simulink model "Controller"  (R2018b)
settings: configuration reference "control_config" (kept outside this file)
values from neighbouring files (symbols this model uses):
  CONTROL_EXPORT = Simulink.Parameter(CONTROL_EXPORT_VALUE)    [controller_model_init.m]
  CONTROL_PARAM = Simulink.Parameter(CONTROL_PARAM_VALUE)    [controller_model_init.m]
undefined symbols (not defined in the file or in its folder): actuator_cmd, CONTROL_CONST, CONTROL_PARAM_VALUE, ControlMode, DiscIntNeverNeededParam, phi_cmd, theta_cmd, timestamp, w_cmd
libraries: simulink x38, FMT_Model_Lib x20
(part 2 of 3)

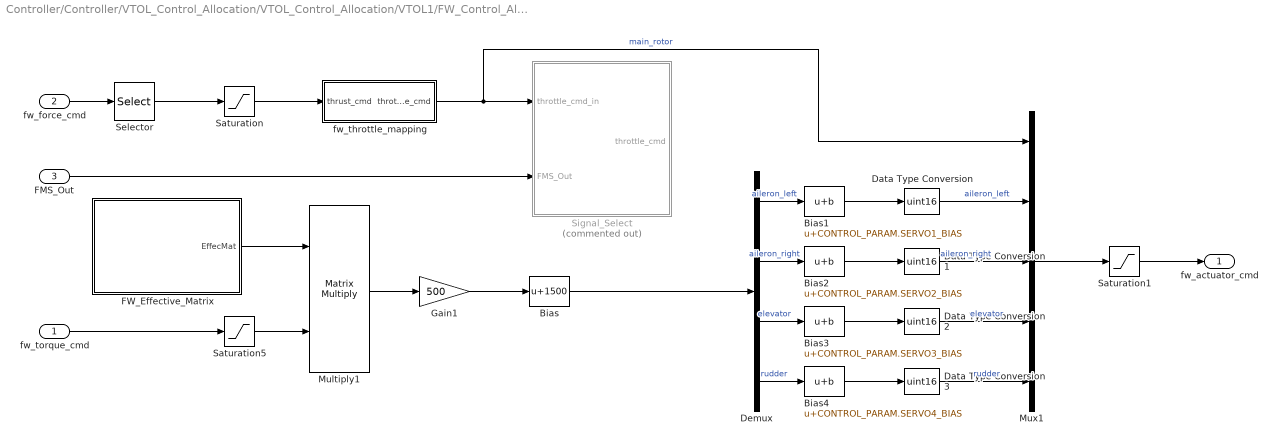
== system Controller/Controller/VTOL_Control_Allocation/VTOL_Control_Allocation/VTOL1/FW_Control_Allocation ==
  fw_torque_cmd : Inport
  fw_force_cmd : Inport  Port=2
  FMS_Out : Inport  Port=3
  Bias : Bias  Bias=1500
  Bias1 : Bias  Bias=CONTROL_PARAM.SERVO1_BIAS
  Bias2 : Bias  Bias=CONTROL_PARAM.SERVO2_BIAS
  Bias3 : Bias  Bias=CONTROL_PARAM.SERVO3_BIAS
  Bias4 : Bias  Bias=CONTROL_PARAM.SERVO4_BIAS
  Data Type Conversion{,1..3} (4 alike) : DataTypeConversion  OutDataTypeStr=uint16
  Demux : Demux
  FW_Effective_Matrix : Subsystem
  Gain1 : Gain  Gain=500  OutDataTypeStr=Inherit: Same as input  ParamDataTypeStr=Inherit: Same as input
  Multiply1 : Product  Multiplication=Matrix(*)  OutDataTypeStr=Inherit: Same as first input
  Mux1 : Mux  Inputs=5
  Saturation : Saturate  UpperLimit=1  LowerLimit=0
  Saturation1 : Saturate  UpperLimit=up_limit  LowerLimit=lo_limit  OutDataTypeStr=uint16
  Saturation5 : Saturate  UpperLimit=1  LowerLimit=-1
  Selector : Selector  InputPortWidth=3  IndexOptions=Index vector (dialog)  Indices=1  OutputSizes=1
  Signal_Select : Subsystem  Commented=on
  fw_throttle_mapping : Subsystem
  fw_actuator_cmd : Outport
  wires:
  Data Type Conversion/1 -> Mux1/2  "aileron_left"
  Gain1/1 -> Bias/1
  Saturation5/1 -> Multiply1/2
  Saturation/1 -> fw_throttle_mapping/1(thrust_cmd)
  Selector/1 -> Saturation/1
  Data Type Conversion1/1 -> Mux1/3  "aileron_right"
  Data Type Conversion3/1 -> Mux1/5  "rudder"
  FW_Effective_Matrix/1(EffecMat) -> Multiply1/1
  fw_force_cmd/1 -> Selector/1
  Data Type Conversion2/1 -> Mux1/4  "elevator"
  Mux1/1 -> Saturation1/1
  Multiply1/1 -> Gain1/1
  fw_torque_cmd/1 -> Saturation5/1
  fw_throttle_mapping/1(throttle_cmd) -> Mux1/1, Signal_Select/1(throttle_cmd_in)  "main_rotor"
  FMS_Out/1 -> Signal_Select/2(FMS_Out)
  Bias/1 -> Demux/1
  Saturation1/1 -> fw_actuator_cmd/1
  Bias2/1 -> Data Type Conversion1/1
  Bias1/1 -> Data Type Conversion/1
  Bias3/1 -> Data Type Conversion2/1
  Bias4/1 -> Data Type Conversion3/1
  Demux/1 -> Bias1/1  "aileron_left"
  Demux/2 -> Bias2/1  "aileron_right"
  Demux/3 -> Bias3/1  "elevator"
  Demux/4 -> Bias4/1  "rudder"

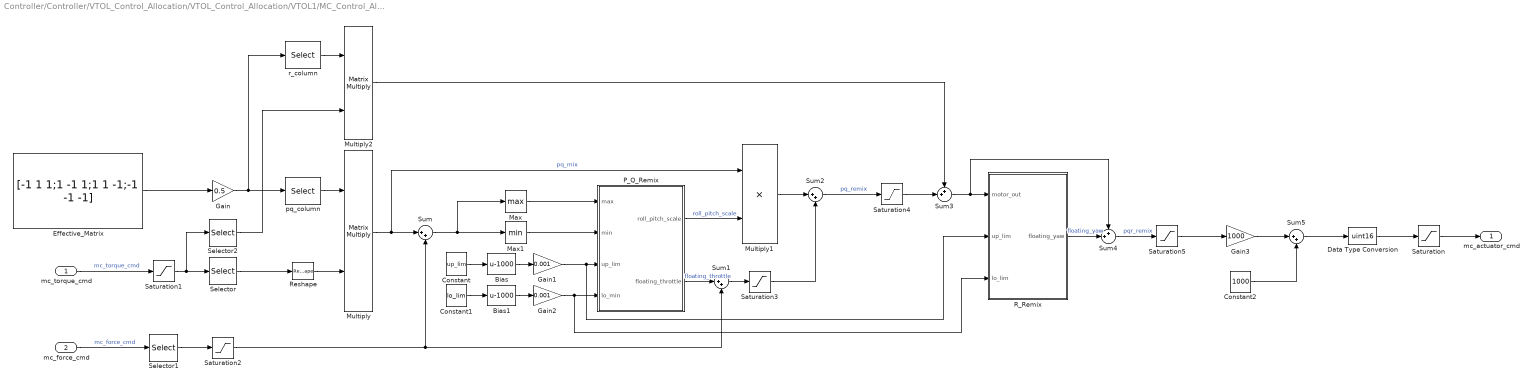
== system Controller/Controller/VTOL_Control_Allocation/VTOL_Control_Allocation/VTOL1/MC_Control_Allocation ==
  mc_torque_cmd : Inport
  mc_force_cmd : Inport  Port=2
  Bias : Bias  Bias=-1000
  Bias1 : Bias  Bias=-1000
  Constant : Constant  Value=up_lim  OutDataTypeStr=single
  Constant1 : Constant  Value=lo_lim  OutDataTypeStr=single
  Constant2 : Constant  Value=1000  OutDataTypeStr=uint32
  Data Type Conversion : DataTypeConversion  OutDataTypeStr=uint16
  Effective_Matrix : Constant  Value=[-1 1 1;1 -1 1;1 1 -1;-1 -1 -1]  OutDataTypeStr=single
  Gain : Gain  Gain=0.5
  Gain1 : Gain  Gain=0.001
  Gain2 : Gain  Gain=0.001
  Gain3 : Gain  Gain=1000  OutDataTypeStr=uint32
  Max : MinMax  Function=max
  Max1 : MinMax
  Multiply : Product  Multiplication=Matrix(*)  OutDataTypeStr=single
  Multiply1 : Product  OutDataTypeStr=single
  Multiply2 : Product  Multiplication=Matrix(*)  OutDataTypeStr=single
  P_Q_Remix : Subsystem
  R_Remix : MATLAB Function  TreatAsAtomicUnit=on
  Reshape : Reshape  OutputDimensionality=Column vector (2-D)
  Saturation : Saturate  UpperLimit=up_lim  LowerLimit=lo_lim
  Saturation1 : Saturate  UpperLimit=1  LowerLimit=-1
  Saturation{2..5} (4 alike) : Saturate  UpperLimit=1  LowerLimit=0
  Selector : Selector  InputPortWidth=3  IndexOptions=Index vector (dialog)  Indices=[1 2]  OutputSizes=1
  Selector1 : Selector  InputPortWidth=3  IndexOptions=Index vector (dialog)  Indices=3  OutputSizes=1
  Selector2 : Selector  InputPortWidth=3  IndexOptions=Index vector (dialog)  Indices=3  OutputSizes=1
  Sum{,1..2,5} (4 alike) : Sum  Inputs=|++
  Sum3 : Sum  Inputs=++|
  Sum4 : Sum  Inputs=++|
  pq_column : Selector  NumberOfDimensions=2  InputPortWidth=3  IndexOptions=Index vector (dialog),Index vector (dialog)  Indices=[1:4],[1 2]  OutputSizes=1,1
  r_column : Selector  NumberOfDimensions=2  InputPortWidth=3  IndexOptions=Index vector (dialog),Index vector (dialog)  Indices=[1:4],3  OutputSizes=1,1
  mc_actuator_cmd : Outport
  wires:
  Multiply/1 -> Multiply1/1, Sum/1  "pq_mix"
  Effective_Matrix/1 -> Gain/1
  mc_force_cmd/1 -> Selector1/1  "mc_force_cmd"
  Sum/1 -> Max/1, Max1/1
  Saturation/1 -> mc_actuator_cmd/1
  Reshape/1 -> Multiply/2
  Selector/1 -> Reshape/1
  Saturation1/1 -> Selector2/1, Selector/1
  Selector1/1 -> Saturation2/1
  pq_column/1 -> Multiply/1
  Max/1 -> P_Q_Remix/1(max)
  Max1/1 -> P_Q_Remix/2(min)
  Gain/1 -> r_column/1, pq_column/1
  P_Q_Remix/2(floating_throttle) -> Sum1/1  "floating_throttle"
  Sum1/1 -> Saturation3/1
  P_Q_Remix/1(roll_pitch_scale) -> Multiply1/2  "roll_pitch_scale"
  Multiply1/1 -> Sum2/1
  Saturation3/1 -> Sum2/2
  Sum2/1 -> Saturation4/1  "pq_remix"
  r_column/1 -> Multiply2/1
  Selector2/1 -> Multiply2/2
  Multiply2/1 -> Sum3/1
  Saturation4/1 -> Sum3/2
  Sum3/1 -> Sum4/1, R_Remix/1(motor_out)
  Constant/1 -> Bias/1
  Constant1/1 -> Bias1/1
  R_Remix/1(floating_yaw) -> Sum4/2  "floating_yaw"
  Sum4/1 -> Saturation5/1  "pqr_remix"
  Data Type Conversion/1 -> Saturation/1
  Bias/1 -> Gain1/1
  Gain1/1 -> P_Q_Remix/3(up_lim), R_Remix/2(up_lim)
  Bias1/1 -> Gain2/1
  Gain2/1 -> P_Q_Remix/4(lo_min), R_Remix/3(lo_lim)
  mc_torque_cmd/1 -> Saturation1/1  "mc_torque_cmd"
  Sum5/1 -> Data Type Conversion/1
  Saturation5/1 -> Gain3/1
  Gain3/1 -> Sum5/1
  Constant2/1 -> Sum5/2
  Saturation2/1 -> Sum1/2, Sum/2

== system Controller/Controller/VTOL_Control_Allocation/VTOL_Control_Allocation/VTOL1/MC_Control_Allocation1 ==
  mc_torque_cmd : Inport
  mc_force_cmd : Inport  Port=2
  Add : Sum  OutDataTypeStr=uint16
  Effective_Matrix : Constant  Value=[-sqrt(2) sqrt(2) 1;sqrt(2) -sqrt(2) 1;sqrt(2) sqrt(2) -1;-sqrt(2) -sqrt(2) -1]  OutDataTypeStr=single
  Gain : Gain  Gain=1000  OutDataTypeStr=Inherit: Same as input
  Multiply : Product  Multiplication=Matrix(*)  OutDataTypeStr=Inherit: Same as first input
  Saturation : Saturate  UpperLimit=1900  LowerLimit=1100
  Saturation1 : Saturate  UpperLimit=1  LowerLimit=-1
  Saturation2 : Saturate  UpperLimit=1  LowerLimit=0
  Selector1 : Selector  InputPortWidth=3  IndexOptions=Index vector (dialog)  Indices=3  OutputSizes=1
  throttle_mapping : Subsystem
  mc_actuator_cmd : Outport
  wires:
  throttle_mapping/1(throttle_cmd) -> Add/2
  Saturation2/1 -> throttle_mapping/1(thrust_cmd)
  Multiply/1 -> Gain/1  "tt2"
  mc_torque_cmd/1 -> Saturation1/1
  Saturation1/1 -> Multiply/2
  Selector1/1 -> Saturation2/1
  Gain/1 -> Add/1
  Effective_Matrix/1 -> Multiply/1
  mc_force_cmd/1 -> Selector1/1
  Add/1 -> Saturation/1
  Saturation/1 -> mc_actuator_cmd/1

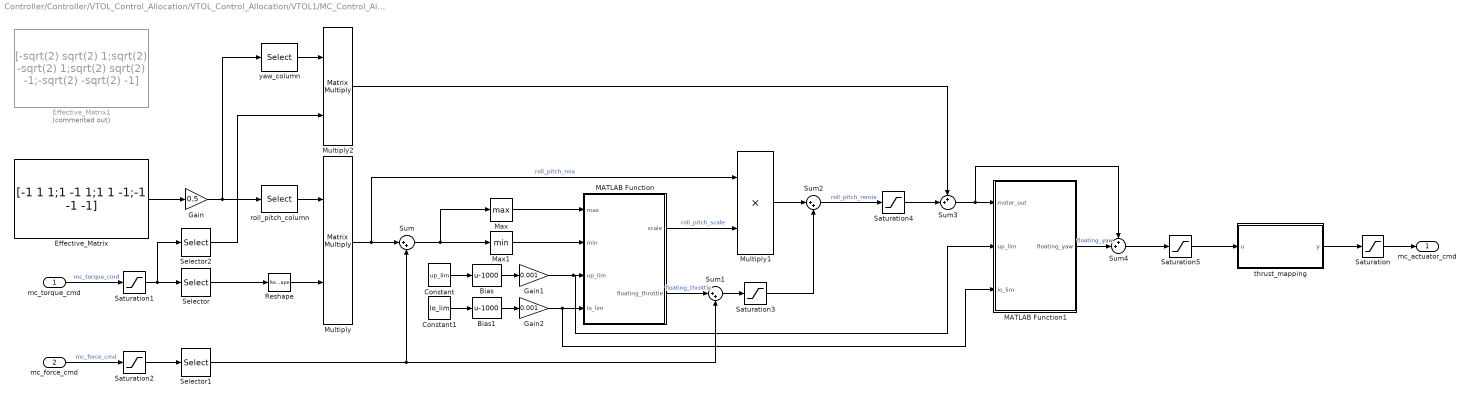
== system Controller/Controller/VTOL_Control_Allocation/VTOL_Control_Allocation/VTOL1/MC_Control_Allocation2 ==
  mc_torque_cmd : Inport
  mc_force_cmd : Inport  Port=2
  Bias : Bias  Bias=-1000
  Bias1 : Bias  Bias=-1000
  Constant : Constant  Value=up_lim  OutDataTypeStr=single
  Constant1 : Constant  Value=lo_lim  OutDataTypeStr=single
  Effective_Matrix : Constant  Value=[-1 1 1;1 -1 1;1 1 -1;-1 -1 -1]  OutDataTypeStr=single
  Effective_Matrix1 : Constant  Commented=on  Value=[-sqrt(2) sqrt(2) 1;sqrt(2) -sqrt(2) 1;sqrt(2) sqrt(2) -1;-sqrt(2) -sqrt(2) -1]  OutDataTypeStr=single
  Gain : Gain  Gain=0.5
  Gain1 : Gain  Gain=0.001
  Gain2 : Gain  Gain=0.001
  MATLAB Function : MATLAB Function  TreatAsAtomicUnit=on
  MATLAB Function1 : MATLAB Function  TreatAsAtomicUnit=on
  Max : MinMax  Function=max
  Max1 : MinMax
  Multiply : Product  Multiplication=Matrix(*)  OutDataTypeStr=Inherit: Same as first input
  Multiply1 : Product
  Multiply2 : Product  Multiplication=Matrix(*)  OutDataTypeStr=Inherit: Same as first input
  Reshape : Reshape  OutputDimensionality=Column vector (2-D)
  Saturation : Saturate  UpperLimit=up_lim  LowerLimit=lo_lim
  Saturation1 : Saturate  UpperLimit=1  LowerLimit=-1
  Saturation{2..5} (4 alike) : Saturate  UpperLimit=1  LowerLimit=0
  Selector : Selector  InputPortWidth=3  IndexOptions=Index vector (dialog)  Indices=[1 2]  OutputSizes=1
  Selector1 : Selector  InputPortWidth=3  IndexOptions=Index vector (dialog)  Indices=3  OutputSizes=1
  Selector2 : Selector  InputPortWidth=3  IndexOptions=Index vector (dialog)  Indices=3  OutputSizes=1
  Sum : Sum  Inputs=|++
  Sum1 : Sum  Inputs=|++
  Sum2 : Sum  Inputs=|++
  Sum3 : Sum  Inputs=++|
  Sum4 : Sum  Inputs=++|
  roll_pitch_column : Selector  NumberOfDimensions=2  InputPortWidth=3  IndexOptions=Index vector (dialog),Index vector (dialog)  Indices=[1:4],[1 2]  OutputSizes=1,1
  thrust_mapping : Subsystem
  yaw_column : Selector  NumberOfDimensions=2  InputPortWidth=3  IndexOptions=Index vector (dialog),Index vector (dialog)  Indices=[1:4],3  OutputSizes=1,1
  mc_actuator_cmd : Outport
  wires:
  Multiply/1 -> Multiply1/1, Sum/1  "roll_pitch_mix"
  Effective_Matrix/1 -> Gain/1
  mc_force_cmd/1 -> Saturation2/1  "mc_force_cmd"
  Sum/1 -> Max/1, Max1/1
  Saturation/1 -> mc_actuator_cmd/1
  Reshape/1 -> Multiply/2
  Selector/1 -> Reshape/1
  Saturation1/1 -> Selector2/1, Selector/1
  Selector1/1 -> Sum1/2, Sum/2
  roll_pitch_column/1 -> Multiply/1
  Max/1 -> MATLAB Function/1(max)
  Max1/1 -> MATLAB Function/2(min)
  Gain/1 -> yaw_column/1, roll_pitch_column/1
  MATLAB Function/2(floating_throttle) -> Sum1/1  "floating_throttle"
  Sum1/1 -> Saturation3/1
  MATLAB Function/1(scale) -> Multiply1/2  "roll_pitch_scale"
  Multiply1/1 -> Sum2/1
  Saturation3/1 -> Sum2/2
  Sum2/1 -> Saturation4/1  "roll_pitch_remix"
  yaw_column/1 -> Multiply2/1
  Selector2/1 -> Multiply2/2
  Multiply2/1 -> Sum3/1
  Saturation4/1 -> Sum3/2
  Sum3/1 -> Sum4/1, MATLAB Function1/1(motor_out)
  Constant/1 -> Bias/1
  Constant1/1 -> Bias1/1
  MATLAB Function1/1(floating_yaw) -> Sum4/2  "floating_yaw"
  Sum4/1 -> Saturation5/1
  Saturation5/1 -> thrust_mapping/1(u)
  thrust_mapping/1(y) -> Saturation/1
  Bias/1 -> Gain1/1
  Gain1/1 -> MATLAB Function/3(up_lim), MATLAB Function1/2(up_lim)
  Bias1/1 -> Gain2/1
  Gain2/1 -> MATLAB Function1/3(lo_lim), MATLAB Function/4(lo_lim)
  Saturation2/1 -> Selector1/1
  mc_torque_cmd/1 -> Saturation1/1  "mc_torque_cmd"

== system Controller/Controller/VTOL_Control_Allocation/VTOL_Control_Allocation/VTOL1/actuator_cmd_routing ==
  cmd_in : Inport
  status : Inport  Port=2
  Disarm : Subsystem
  Multiport Switch : MultiPortSwitch  DataPortForDefault=Additional data port  DiagnosticForDefault=None
  Standby : Subsystem
  cmd_out : Outport
  wires:
  Multiport Switch/1 -> cmd_out/1
  status/1 -> Multiport Switch/1
  cmd_in/1 -> Multiport Switch/4
  Disarm/1(actuator_cmd) -> Multiport Switch/5, Multiport Switch/2
  Standby/1(actuator_cmd) -> Multiport Switch/3

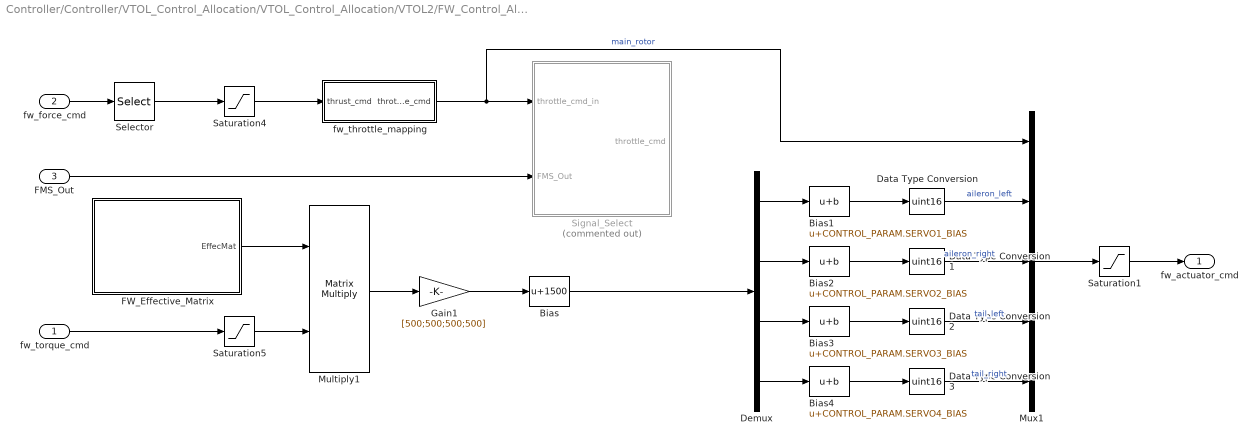
== system Controller/Controller/VTOL_Control_Allocation/VTOL_Control_Allocation/VTOL2/FW_Control_Allocation ==
  fw_torque_cmd : Inport
  fw_force_cmd : Inport  Port=2
  FMS_Out : Inport  Port=3
  Bias : Bias  Bias=1500
  Bias1 : Bias  Bias=CONTROL_PARAM.SERVO1_BIAS
  Bias2 : Bias  Bias=CONTROL_PARAM.SERVO2_BIAS
  Bias3 : Bias  Bias=CONTROL_PARAM.SERVO3_BIAS
  Bias4 : Bias  Bias=CONTROL_PARAM.SERVO4_BIAS
  Data Type Conversion{,1..3} (4 alike) : DataTypeConversion  OutDataTypeStr=uint16
  Demux : Demux
  FW_Effective_Matrix : Subsystem
  Gain1 : Gain  Gain=[500;500;500;500]  OutDataTypeStr=Inherit: Same as input  ParamDataTypeStr=Inherit: Same as input
  Multiply1 : Product  Multiplication=Matrix(*)  OutDataTypeStr=Inherit: Same as first input
  Mux1 : Mux  Inputs=5
  Saturation1 : Saturate  UpperLimit=1950  LowerLimit=1050  OutDataTypeStr=uint16
  Saturation4 : Saturate  UpperLimit=1  LowerLimit=0
  Saturation5 : Saturate  UpperLimit=1  LowerLimit=-1
  Selector : Selector  InputPortWidth=3  IndexOptions=Index vector (dialog)  Indices=1  OutputSizes=1
  Signal_Select : Subsystem  Commented=on
  fw_throttle_mapping : Subsystem
  fw_actuator_cmd : Outport
  wires:
  Demux/1 -> Bias1/1
  Gain1/1 -> Bias/1
  Saturation5/1 -> Multiply1/2
  Saturation4/1 -> fw_throttle_mapping/1(thrust_cmd)
  Selector/1 -> Saturation4/1
  Demux/2 -> Bias2/1
  Demux/4 -> Bias4/1
  FW_Effective_Matrix/1(EffecMat) -> Multiply1/1
  fw_force_cmd/1 -> Selector/1
  Demux/3 -> Bias3/1
  Mux1/1 -> Saturation1/1
  Multiply1/1 -> Gain1/1
  fw_torque_cmd/1 -> Saturation5/1
  fw_throttle_mapping/1(throttle_cmd) -> Mux1/1, Signal_Select/1(throttle_cmd_in)  "main_rotor"
  FMS_Out/1 -> Signal_Select/2(FMS_Out)
  Bias/1 -> Demux/1
  Saturation1/1 -> fw_actuator_cmd/1
  Bias1/1 -> Data Type Conversion/1
  Bias2/1 -> Data Type Conversion1/1
  Bias3/1 -> Data Type Conversion2/1
  Bias4/1 -> Data Type Conversion3/1
  Data Type Conversion/1 -> Mux1/2  "aileron_left"
  Data Type Conversion1/1 -> Mux1/3  "aileron_right"
  Data Type Conversion2/1 -> Mux1/4  "tail_left"
  Data Type Conversion3/1 -> Mux1/5  "tail_right"

== system Controller/Controller/VTOL_Control_Allocation/VTOL_Control_Allocation/VTOL2/MC_Control_Allocation ==
  mc_torque_cmd : Inport
  mc_force_cmd : Inport  Port=2
  Add : Sum  OutDataTypeStr=uint16
  Effective_Matrix : Constant  Value=[-sqrt(2) sqrt(2) 1;sqrt(2) -sqrt(2) 1;sqrt(2) sqrt(2) -1;-sqrt(2) -sqrt(2) -1]  OutDataTypeStr=single
  Gain : Gain  Gain=1000  OutDataTypeStr=Inherit: Same as input
  Multiply : Product  Multiplication=Matrix(*)  OutDataTypeStr=Inherit: Same as first input
  Saturation : Saturate  UpperLimit=1950  LowerLimit=1050
  Saturation1 : Saturate  UpperLimit=1  LowerLimit=-1
  Saturation2 : Saturate  UpperLimit=1  LowerLimit=0
  Selector1 : Selector  InputPortWidth=3  IndexOptions=Index vector (dialog)  Indices=3  OutputSizes=1
  throttle_mapping : Subsystem
  mc_actuator_cmd : Outport
  wires:
  throttle_mapping/1(throttle_cmd) -> Add/2
  Saturation2/1 -> throttle_mapping/1(thrust_cmd)
  Multiply/1 -> Gain/1
  mc_torque_cmd/1 -> Saturation1/1
  Saturation1/1 -> Multiply/2
  Selector1/1 -> Saturation2/1
  Gain/1 -> Add/1
  Effective_Matrix/1 -> Multiply/1
  mc_force_cmd/1 -> Selector1/1
  Add/1 -> Saturation/1
  Saturation/1 -> mc_actuator_cmd/1

== system Controller/Controller/VTOL_Control_Allocation/VTOL_Control_Allocation/VTOL2/actuator_cmd_routing ==
  cmd_in : Inport
  status : Inport  Port=2
  Disarm : Subsystem
  Multiport Switch : MultiPortSwitch  DataPortForDefault=Additional data port  DiagnosticForDefault=None
  Standby : Subsystem
  cmd_out : Outport
  wires:
  Multiport Switch/1 -> cmd_out/1
  Standby/1(actuator_cmd) -> Multiport Switch/3
  status/1 -> Multiport Switch/1
  cmd_in/1 -> Multiport Switch/4
  Disarm/1(actuator_cmd) -> Multiport Switch/5, Multiport Switch/2

== system Controller/Controller/FW_Controller/Aux_MC_Controller/Attitude_Controller/Inner_Loop/Rate_Controller ==
  rate_cmd_radPs : Inport
  INS_Out : Inport  Port=2
  reset : Inport  Port=3
  Error : Subsystem
  PID_Controller : Subsystem
  rate_dot_cmd_B : Outport
  wires:
  INS_Out/1 -> Error/2(INS_Out)
  Error/1(rate_err_radPs) -> PID_Controller/1(rate_err_radPs)
  rate_cmd_radPs/1 -> Error/1(rate_cmd_radPs)
  reset/1 -> PID_Controller/2(reset)
  PID_Controller/1(rate_dot_cmd_B) -> rate_dot_cmd_B/1

== system Controller/Controller/FW_Controller/Aux_MC_Controller/Attitude_Controller/Inner_Loop/Signal_Convert ==
  FMS_Out : Inport
  euler_rate_cmd : Inport  Port=2
  INS_Out : Inport  Port=3
  Bus Selector2 : BusSelector  OutputSignals=psi_rate_cmd
  Bus Selector3 : BusSelector  OutputSignals=phi,theta
  Demux : Demux  Outputs=3
  Euler To Angle Rate : FMT_Model_Lib/Math/Euler To Angle Rate
      settings: SourceProductName=FMT Toolbox
  Mux : Mux  Inputs=3
  Mux1 : Mux  Inputs=2
  Mux2 : Mux  Inputs=2
  Saturation2 : Saturate  UpperLimit=CONTROL_PARAM.MC_R_CMD_LIM  LowerLimit=-CONTROL_PARAM.MC_R_CMD_LIM
  Saturation3 : Saturate  UpperLimit=CONTROL_PARAM.MC_P_Q_CMD_LIM  LowerLimit=-CONTROL_PARAM.MC_P_Q_CMD_LIM
  Saturation4 : Saturate  UpperLimit=CONTROL_PARAM.MC_P_Q_CMD_LIM  LowerLimit=-CONTROL_PARAM.MC_P_Q_CMD_LIM
  rate_cmd_radPs : Outport
  wires:
  Bus Selector3/1 -> Mux2/1  "<phi>"
  Mux2/1 -> Euler To Angle Rate/1
  Bus Selector3/2 -> Mux2/2  "<theta>"
  Bus Selector2/1 -> Mux1/2  "<psi_rate_cmd>"
  Mux1/1 -> Euler To Angle Rate/2  "aux_euler_rate"
  FMS_Out/1 -> Bus Selector2/1
  INS_Out/1 -> Bus Selector3/1
  euler_rate_cmd/1 -> Mux1/1
  Demux/3 -> Saturation2/1
  Saturation3/1 -> Mux/1
  Saturation4/1 -> Mux/2
  Euler To Angle Rate/1 -> Demux/1  "aux_angle_rate"
  Demux/2 -> Saturation4/1
  Mux/1 -> rate_cmd_radPs/1
  Saturation2/1 -> Mux/3
  Demux/1 -> Saturation3/1

== system Controller/Controller/FW_Controller/Aux_MC_Controller/Attitude_Controller/Outter_Loop/Attitude_Controller ==
  att_cmd_rad : Inport
  INS_Out : Inport  Port=2
  Error : Subsystem
  Sqrt_Root_Controller : Subsystem
  euler_rate_cmd_radPs : Outport
  wires:
  INS_Out/1 -> Error/2(INS_Out)
  Sqrt_Root_Controller/1(euler_rate_cmd_radPs) -> euler_rate_cmd_radPs/1
  att_cmd_rad/1 -> Error/1(att_cmd)
  Error/1(euler_err_rad) -> Sqrt_Root_Controller/1(euler_err_rad)

== system Controller/Controller/FW_Controller/Aux_MC_Controller/Aux_Commander/Commander/Phi_Commander ==
  FMS_Out : Inport
  aux_cmd : Inport  Port=2
  Altitude : simulink/Logic and Bit Operations/Compare To Constant  relop=<=  const=uint8(ControlMode.ALTCTL)  OutDataTypeStr=boolean
  Bus Selector : BusSelector  OutputSignals=phi_cmd,ctrl_mode
  Bus Selector1 : BusSelector  OutputSignals=fw_phi_cmd
  Switch : Switch  Criteria=u2 > Threshold
  phi_cmd : Outport  VectorParamsAs1DForOutWhenUnconnected=on
  wires:
  Bus Selector/2 -> Altitude/1  "<ctrl_mode>"
  Bus Selector/1 -> Switch/1  "<phi_cmd>"
  FMS_Out/1 -> Bus Selector/1
  Altitude/1 -> Switch/2
  aux_cmd/1 -> Bus Selector1/1
  Bus Selector1/1 -> Switch/3  "<fw_phi_cmd>"
  Switch/1 -> phi_cmd/1

== system Controller/Controller/FW_Controller/Aux_MC_Controller/Aux_Commander/Commander/Theta_Commander ==
  FMS_Out : Inport
  aux_cmd : Inport  Port=2
  Bus Selector : BusSelector  OutputSignals=theta_cmd,ctrl_mode
  Bus Selector1 : BusSelector  OutputSignals=fw_theta_cmd
  Stabilize : simulink/Logic and Bit Operations/Compare To Constant  relop=<=  const=uint8(ControlMode.Stabilize)  OutDataTypeStr=boolean
  Switch : Switch  Criteria=u2 > Threshold
  theta_cmd : Outport  VectorParamsAs1DForOutWhenUnconnected=on
  wires:
  Bus Selector/2 -> Stabilize/1  "<ctrl_mode>"
  Bus Selector/1 -> Switch/1  "<theta_cmd>"
  FMS_Out/1 -> Bus Selector/1
  Stabilize/1 -> Switch/2
  aux_cmd/1 -> Bus Selector1/1
  Bus Selector1/1 -> Switch/3  "<fw_theta_cmd>"
  Switch/1 -> theta_cmd/1

== system Controller/Controller/FW_Controller/Aux_MC_Controller/Aux_Commander/Commander/W_Commander ==
  FMS_Out : Inport
  Bus Selector : BusSelector  OutputSignals=ctrl_mode,w_cmd
  Stabilize : simulink/Logic and Bit Operations/Compare To Constant  relop=<=  const=uint8(ControlMode.Stabilize)  OutDataTypeStr=boolean
  Switch : Switch  Criteria=u2 > Threshold
  Zero : Constant  Value=0  OutDataTypeStr=single
  w_cmd : Outport  VectorParamsAs1DForOutWhenUnconnected=on
  wires:
  Bus Selector/1 -> Stabilize/1  "<ctrl_mode>"
  Bus Selector/2 -> Switch/3  "<w_cmd>"
  FMS_Out/1 -> Bus Selector/1
  Stabilize/1 -> Switch/2
  Zero/1 -> Switch/1
  Switch/1 -> w_cmd/1

== system Controller/Controller/FW_Controller/Aux_MC_Controller/Vertical_Control/Veloxity_Z_Controller/Boosted_Throttle ==
  thrust_cmd : Inport
  INS_Out : Inport  Port=2
  Bus Selector : BusSelector  OutputSignals=phi,theta
  Constant : Constant  OutDataTypeStr=single
  Cos : Trigonometry  Operator=cos
  Cos1 : Trigonometry  Operator=cos
  Divide : Product  Inputs=*/
  Gain : Gain  Gain=2
  Multiply : Product
  Multiply1 : Product  Inputs=3
  Saturation : Saturate  UpperLimit=1  LowerLimit=0
  Saturation1 : Saturate  UpperLimit=1  LowerLimit=0.5
  boosted_thrust : Outport
  wires:
  INS_Out/1 -> Bus Selector/1
  Bus Selector/1 -> Cos/1  "<phi>"
  Bus Selector/2 -> Cos1/1  "<theta>"
  Cos/1 -> Multiply/1
  Cos1/1 -> Multiply/2
  Multiply/1 -> Saturation1/1, Gain/1
  Gain/1 -> Saturation/1
  Saturation/1 -> Multiply1/3  "inverted_factor"
  Constant/1 -> Divide/1
  Divide/1 -> Multiply1/2  "boost_factor"
  Saturation1/1 -> Divide/2
  thrust_cmd/1 -> Multiply1/1
  Multiply1/1 -> boosted_thrust/1

== system Controller/Controller/FW_Controller/Aux_MC_Controller/Vertical_Control/Veloxity_Z_Controller/Error ==
  FMS_Out : Inport
  INS_Out : Inport  Port=2
  Bus Selector1 : BusSelector  OutputSignals=vd
  Bus Selector2 : BusSelector  OutputSignals=w_cmd
  Gain : Gain  Gain=-1  OutDataTypeStr=Inherit: Same as input
  Signal Copy1 : SignalConversion  OverrideOpt=off
  Sum1 : Sum  Inputs=|+-
  TD : Subsystem
  vu_cmd_C_mPs : Outport
  wires:
  INS_Out/1 -> Bus Selector1/1
  Bus Selector2/1 -> TD/1(v)  "<w_cmd>"
  Bus Selector1/1 -> Signal Copy1/1  "<vd>"
  Gain/1 -> vu_cmd_C_mPs/1
  Sum1/1 -> Gain/1  "w_error_C_mPs"
  FMS_Out/1 -> Bus Selector2/1
  TD/1(v1) -> Sum1/1  "w_cmd_C_mPs"
  Signal Copy1/1 -> Sum1/2  "w_est_C_mPs"

== system Controller/Controller/FW_Controller/Aux_MC_Controller/Vertical_Control/Veloxity_Z_Controller/PID_Controller ==
  vu_cmd_C_mPs : Inport
  reset : Inport  Port=2
  Add : Sum  Inputs=+++
  D_Control : Subsystem  mask{kd=CONTROL_PARAM.MC_VEL_Z_D, max_d=CONTROL_PARAM.MC_VEL_Z_D_MAX, min_d=CONTROL_PARAM.MC_VEL_Z_D_MIN}
  I_Control : Subsystem  mask{ki=CONTROL_PARAM.MC_VEL_Z_I, max_i=CONTROL_PARAM.MC_VEL_Z_I_MAX, min_i=CONTROL_PARAM.MC_VEL_Z_I_MIN}
  P_Control : Subsystem  mask{kp=CONTROL_PARAM.MC_VEL_Z_P}
  thrust_cmd : Outport
  wires:
  P_Control/1(p_out) -> Add/1  "thrust_p_out"
  I_Control/1(i_out) -> Add/2  "thrust_i_out"
  Add/1 -> thrust_cmd/1
  vu_cmd_C_mPs/1 -> D_Control/1(err), I_Control/1(err), P_Control/1(err)
  D_Control/1(d_out) -> Add/3  "thrust_d_out"
  reset/1 -> I_Control/2(reset), D_Control/2(reset)

== system Controller/Controller/FW_Controller/FW_Controller/Attitude_Control/Innerloop_Rate_Control/PI_Control ==
  error : Inport
  reset : Inport  Port=2
  Add1 : Sum
  I_Control : Subsystem  mask{p_ki=CONTROL_PARAM.FW_ROLL_RATE_I, q_ki=CONTROL_PARAM.FW_PITCH_RATE_I, r_ki=CONTROL_PARAM.FW_YAW_RATE_I, max_i=CONTROL_PARAM.FW_RATE_I_MAX, min_i=CONTROL_PARAM.FW_RATE_I_MIN}
  P_Control : Subsystem  mask{p_kp=CONTROL_PARAM.FW_ROLL_RATE_P, q_kp=CONTROL_PARAM.FW_PITCH_RATE_P, r_kp=CONTROL_PARAM.FW_YAW_RATE_P}
  pi_out : Outport
  wires:
  Add1/1 -> pi_out/1
  I_Control/1(i_out) -> Add1/2  "i_out"
  error/1 -> P_Control/1(err), I_Control/1(err)
  P_Control/1(p_out) -> Add1/1  "p_out"
  reset/1 -> I_Control/2(reset)

== system Controller/Controller/FW_Controller/FW_Controller/Attitude_Control/Innerloop_Rate_Control/PI_scaler ==
  VT : Inport
  Divide : Product  Inputs=*/
  Saturation : Saturate  UpperLimit=1  LowerLimit=0
  Square : Math  Operator=square  SaturateOnIntegerOverflow=on
  Square1 : Math  Operator=square  SaturateOnIntegerOverflow=on
  trim_speed : Constant  Value=CONTROL_PARAM.FW_AIRSPEED_TRIM
  PI_scale : Outport
  wires:
  Square1/1 -> Divide/2
  trim_speed/1 -> Square/1
  Square/1 -> Divide/1
  VT/1 -> Square1/1
  Divide/1 -> Saturation/1
  Saturation/1 -> PI_scale/1

== system Controller/Controller/FW_Controller/FW_Controller/Attitude_Control/Innerloop_Rate_Control/VT_scaler ==
  VT : Inport
  Divide : Product  Inputs=*/
  Saturation : Saturate  UpperLimit=1  LowerLimit=0
  trim_speed : Constant  Value=CONTROL_PARAM.FW_AIRSPEED_TRIM
  FF_scale : Outport
  wires:
  trim_speed/1 -> Divide/1
  VT/1 -> Divide/2
  Divide/1 -> Saturation/1
  Saturation/1 -> FF_scale/1

== system Controller/Controller/FW_Controller/FW_Controller/Attitude_Control/Outloop_Angle_Control/Attitude_Controller ==
  att_cmd : Inport
  INS_Out : Inport  Port=2
  Error : Subsystem
  P_Controller : Subsystem
  phi_theta_rate_cmd : Outport
  wires:
  INS_Out/1 -> Error/2(INS_Out)
  P_Controller/1(u) -> phi_theta_rate_cmd/1
  att_cmd/1 -> Error/1(att_cmd)
  Error/1(euler_err_rad) -> P_Controller/1(error)

== system Controller/Controller/FW_Controller/FW_Controller/Attitude_Control/Outloop_Angle_Control/Heading_Controller ==
  fw_att_cmd : Inport
  FMS_Out : Inport  Port=2
  VT : Inport  Port=3
  Bus Selector2 : BusSelector  OutputSignals=psi_rate_cmd
  Demux : Demux  Outputs=2
  Saturation : Saturate  UpperLimit=CONTROL_PARAM.FW_YAW_RATE_LIM  LowerLimit=-CONTROL_PARAM.FW_YAW_RATE_LIM
  Sum : Sum  Inputs=++|
  Turning_Coordination : Subsystem
  psi_rate_cmd : Outport
  wires:
  Turning_Coordination/1(psi_rate_sp) -> Sum/2  "fw_psi_rate_sp"
  Sum/1 -> Saturation/1
  FMS_Out/1 -> Bus Selector2/1
  VT/1 -> Turning_Coordination/3(VT)
  Bus Selector2/1 -> Sum/1  "<psi_rate_cmd>"
  fw_att_cmd/1 -> Demux/1
  Demux/1 -> Turning_Coordination/1(phi_sp)
  Demux/2 -> Turning_Coordination/2(theta_sp)
  Saturation/1 -> psi_rate_cmd/1

== system Controller/Controller/FW_Controller/FW_Controller/Attitude_Control/Outloop_Angle_Control/Signal_Select ==
  att_cmd_rad : Inport
  FMS_Out : Inport  Port=2
  Bus Selector : BusSelector  OutputSignals=ctrl_mode
  Bus Selector1 : BusSelector  OutputSignals=phi_cmd
  Bus Selector2 : BusSelector  OutputSignals=ctrl_mode
  Bus Selector3 : BusSelector  OutputSignals=theta_cmd
  Compare To Constant : simulink/Logic and Bit Operations/Compare To Constant  relop===  const=uint8([ControlMode.Stabilize, ControlMode.ALTCTL])  OutDataTypeStr=boolean
  Compare To Constant1 : simulink/Logic and Bit Operations/Compare To Constant  relop===  const=uint8([ControlMode.Stabilize])  OutDataTypeStr=boolean
  Logical Operator : Logic  Operator=OR  Inputs=1  AllPortsSameDT=off  OutDataTypeStr=boolean
  Logical Operator1 : Logic  Operator=OR  Inputs=1  AllPortsSameDT=off  OutDataTypeStr=boolean
  Mux : Mux  Inputs=2
  Selector : Selector  InputPortWidth=2  IndexOptions=Index vector (dialog)  Indices=1  OutputSizes=1
  Selector1 : Selector  InputPortWidth=2  IndexOptions=Index vector (dialog)  Indices=2  OutputSizes=1
  Switch : Switch  Criteria=u2 > Threshold
  Switch1 : Switch  Criteria=u2 > Threshold
  fw_att_cmd : Outport
  wires:
  Compare To Constant/1 -> Logical Operator/1
  att_cmd_rad/1 -> Selector/1, Selector1/1
  Bus Selector/1 -> Compare To Constant/1  "<ctrl_mode>"
  FMS_Out/1 -> Bus Selector2/1, Bus Selector3/1, Bus Selector1/1, Bus Selector/1
  Bus Selector1/1 -> Switch/1  "<phi_cmd>"
  Logical Operator/1 -> Switch/2
  Selector/1 -> Switch/3
  Logical Operator1/1 -> Switch1/2
  Compare To Constant1/1 -> Logical Operator1/1
  Bus Selector2/1 -> Compare To Constant1/1  "<ctrl_mode>"
  Bus Selector3/1 -> Switch1/1  "<theta_cmd>"
  Selector1/1 -> Switch1/3
  Switch/1 -> Mux/1  "phi_cmd"
  Switch1/1 -> Mux/2  "theta_cmd"
  Mux/1 -> fw_att_cmd/1

== system Controller/Controller/FW_Controller/FW_Controller/TECS_Core/path_angle_control/Flight_Path_Angle ==
  note: If velocity is not valid, we use
      | theta as gamma.
  INS_Out : Inport
  gamma_dir : Inport  Port=2
  Add : Sum
  Asin : Trigonometry  Operator=atan
  Bitwise AND : simulink/Logic and Bit Operations/Bitwise Operator  logicop=AND  UseBitMask=on  BitMask=bin2dec('10000')  BitMaskRealWorld=Stored Integer
  Bus Selector1 : BusSelector  OutputSignals=flag,theta
  Bus Selector2 : BusSelector  OutputSignals=vn,ve,vd
  Dead Zone : DeadZone  LowerValue=-0.1  UpperValue=0.1  SaturateOnIntegerOverflow=on
  Divide : Product  Inputs=/*
  Gain : Gain  Gain=-1
  Multiply1 : Product
  Saturation : Saturate  UpperLimit=100  LowerLimit=8
  Saturation1 : Saturate  UpperLimit=pi/4  LowerLimit=-pi/4
  Sqrt : Sqrt  SaturateOnIntegerOverflow=on
  Square : Math  Operator=square  SaturateOnIntegerOverflow=on
  Square1 : Math  Operator=square  SaturateOnIntegerOverflow=on
  Switch : Switch  Criteria=u2 > Threshold  Threshold=1
  gamma : Outport
  wires:
  INS_Out/1 -> Bus Selector1/1, Bus Selector2/1
  Square/1 -> Add/1
  Square1/1 -> Add/2
  Add/1 -> Sqrt/1
  Gain/1 -> Divide/2
  Divide/1 -> Asin/1
  Sqrt/1 -> Saturation/1  "Vg"
  Bus Selector2/1 -> Square/1  "<vn>"
  Bus Selector2/2 -> Square1/1  "<ve>"
  Bus Selector2/3 -> Dead Zone/1  "<vd>"
  Switch/1 -> Multiply1/2
  Bitwise AND/1 -> Switch/2
  Saturation/1 -> Divide/1
  Bus Selector1/1 -> Bitwise AND/1  "<flag>"
  Bus Selector1/2 -> Switch/3  "<theta>"
  Saturation1/1 -> gamma/1
  Dead Zone/1 -> Gain/1
  Asin/1 -> Switch/1
  Multiply1/1 -> Saturation1/1
  gamma_dir/1 -> Multiply1/1

== system Controller/Controller/FW_Controller/FW_Controller/TECS_Core/path_angle_control/Subsystem ==
  INS_Out : Inport
  Bitwise AND : simulink/Logic and Bit Operations/Bitwise Operator  logicop=AND  UseBitMask=on  BitMask=bin2dec('10000')  BitMaskRealWorld=Stored Integer
  Bus Selector1 : BusSelector  OutputSignals=flag
  Bus Selector2 : BusSelector  OutputSignals=vn,ve,vd
  Bus Selector3 : BusSelector  OutputSignals=psi
  Constant : Constant  OutDataTypeStr=single
  Dead Zone : DeadZone  LowerValue=-1  UpperValue=1  SaturateOnIntegerOverflow=on
  Multiply : Product  Multiplication=Matrix(*)
  Mux : Mux  Inputs=3
  Psi To DCM : FMT_Model_Lib/Transformation/Psi To DCM
      settings: SourceProductName=FMT Toolbox
  Selector : Selector  InputPortWidth=3  IndexOptions=Index vector (dialog)  Indices=1  OutputSizes=1
  Sign : Signum
  Switch : Switch  Criteria=u2 > Threshold
  gamma_dir : Outport
  wires:
  Psi To DCM/1 -> Multiply/1
  Bus Selector2/3 -> Mux/3  "<vd>"
  Selector/1 -> Dead Zone/1
  Bus Selector2/2 -> Mux/2  "<ve>"
  Bus Selector3/1 -> Psi To DCM/1  "<psi>"
  Multiply/1 -> Selector/1
  Dead Zone/1 -> Sign/1
  Bus Selector2/1 -> Mux/1  "<vn>"
  Mux/1 -> Multiply/2
  INS_Out/1 -> Bus Selector1/1, Bus Selector2/1, Bus Selector3/1
  Sign/1 -> Switch/1
  Bus Selector1/1 -> Bitwise AND/1  "<flag>"
  Bitwise AND/1 -> Switch/2
  Switch/1 -> gamma_dir/1
  Constant/1 -> Switch/3

== system Controller/Controller/FW_Controller/FW_Controller/TECS_Core/path_angle_control/Target_Flight_Path_Angle ==
  FMS_Out : Inport
  INS_Out : Inport  Port=2
  gamma_dir : Inport  Port=3
  Add : Sum
  Asin : Trigonometry  Operator=atan
  Bitwise AND : simulink/Logic and Bit Operations/Bitwise Operator  logicop=AND  UseBitMask=on  BitMask=bin2dec('10000')  BitMaskRealWorld=Stored Integer
  Bus Selector : BusSelector  OutputSignals=w_cmd
  Bus Selector1 : BusSelector  OutputSignals=vn,ve
  Bus Selector2 : BusSelector  OutputSignals=flag,airspeed
  Divide : Product  Inputs=*/
  Gain : Gain  Gain=-1
  Multiply1 : Product
  Saturation1 : Saturate  UpperLimit=100  LowerLimit=8
  Saturation2 : Saturate  UpperLimit=pi/4  LowerLimit=-pi/4
  Sqrt : Sqrt  SaturateOnIntegerOverflow=on
  Square : Math  Operator=square  SaturateOnIntegerOverflow=on
  Square1 : Math  Operator=square  SaturateOnIntegerOverflow=on
  Switch : Switch  Criteria=u2 > Threshold
  gamma_sp : Outport
  wires:
  FMS_Out/1 -> Bus Selector/1
  Bus Selector/1 -> Gain/1  "<w_cmd>"
  INS_Out/1 -> Bus Selector2/1, Bus Selector1/1
  Divide/1 -> Asin/1
  Square/1 -> Add/1
  Square1/1 -> Add/2
  Add/1 -> Sqrt/1
  Gain/1 -> Divide/1
  Saturation1/1 -> Divide/2
  Bus Selector1/2 -> Square1/1  "<ve>"
  Bus Selector1/1 -> Square/1  "<vn>"
  Sqrt/1 -> Switch/1  "Vg"
  Saturation2/1 -> gamma_sp/1
  Asin/1 -> Multiply1/1
  Multiply1/1 -> Saturation2/1
  gamma_dir/1 -> Multiply1/2
  Bus Selector2/1 -> Bitwise AND/1  "<flag>"
  Switch/1 -> Saturation1/1
  Bitwise AND/1 -> Switch/2
  Bus Selector2/2 -> Switch/3  "<airspeed>"

== system Controller/Controller/FW_Controller/FW_Controller/TECS_Core/pitch_pid_out/D_control ==
  err : Inport
  reset : Inport  Port=2
  DT Filter : FMT_Model_Lib/Filter/DT Filter  fc=10
      settings: SourceProductName=FMT Toolbox
  Gain : Gain  Gain=CONTROL_PARAM.FW_TECS_PITCH_D
  d_out : Outport
  wires:
  reset/1 -> DT Filter/2
  DT Filter/1 -> Gain/1
  Gain/1 -> d_out/1
  err/1 -> DT Filter/1

== system Controller/Controller/FW_Controller/FW_Controller/TECS_Core/pitch_pid_out/I_control ==
  err : Inport
  reset : Inport  Port=2
  " " : DiscreteIntegrator  ExternalReset=level  InitialConditionSource=external  SampleTime=-1  LimitOutput=on  UpperSaturationLimit=CONTROL_PARAM.FW_TECS_PITCH_I_LIM  LowerSaturationLimit=-CONTROL_PARAM.FW_TECS_PITCH_I_LIM  ICPrevOutput=DiscIntNeverNeededParam  ICPrevScaledInput=DiscIntNeverNeededParam
  Gain3 : Gain  Gain=CONTROL_PARAM.FW_TECS_PITCH_I
  Zero1 : Constant  Value=0  OutDataTypeStr=Inherit: Inherit via back propagation
  i_out : Outport
  wires:
  Zero1/1 -> " "/3
  " "/1 -> i_out/1
  Gain3/1 -> " "/1
  err/1 -> Gain3/1
  reset/1 -> " "/2

== system Controller/Controller/FW_Controller/FW_Controller/TECS_Core/thorttle_pid_out/D_control ==
  err : Inport
  reset : Inport  Port=2
  DT Filter : FMT_Model_Lib/Filter/DT Filter  fc=30
      settings: SourceProductName=FMT Toolbox
  Gain : Gain  Gain=CONTROL_PARAM.FW_TECS_THOR_D
  D_out : Outport
  wires:
  reset/1 -> DT Filter/2
  DT Filter/1 -> Gain/1
  err/1 -> DT Filter/1
  Gain/1 -> D_out/1

== system Controller/Controller/FW_Controller/FW_Controller/TECS_Core/thorttle_pid_out/I_control ==
  E_err : Inport
  reset : Inport  Port=2
  " " : DiscreteIntegrator  ExternalReset=level  InitialConditionSource=external  SampleTime=-1  LimitOutput=on  UpperSaturationLimit=1  LowerSaturationLimit=0  ICPrevOutput=DiscIntNeverNeededParam  ICPrevScaledInput=DiscIntNeverNeededParam
  Gain : Gain  Gain=CONTROL_PARAM.FW_TECS_THOR_I
  Zero : Constant  Value=0  OutDataTypeStr=Inherit: Inherit via back propagation
  i_out : Outport
  wires:
  reset/1 -> " "/2
  Zero/1 -> " "/3
  Gain/1 -> " "/1
  E_err/1 -> Gain/1
  " "/1 -> i_out/1

== system Controller/Controller/MC_Controller/Horizontal_Control/Attitude_Controller/Inner_Loop/Rate_Controller ==
  rate_cmd_radPs : Inport
  INS_Out : Inport  Port=2
  reset : Inport  Port=3
  Error : Subsystem
  PID_Controller : Subsystem
  rate_dot_cmd_B : Outport
  wires:
  INS_Out/1 -> Error/2(INS_Out)
  Error/1(rate_err_radPs) -> PID_Controller/1(rate_err_radPs)
  rate_cmd_radPs/1 -> Error/1(rate_cmd_radPs)
  reset/1 -> PID_Controller/2(reset)
  PID_Controller/1(rate_dot_cmd_B) -> rate_dot_cmd_B/1

== system Controller/Controller/MC_Controller/Horizontal_Control/Attitude_Controller/Inner_Loop/Signal_Convert ==
  FMS_Out : Inport
  euler_rate_cmd : Inport  Port=2
  INS_Out : Inport  Port=3
  Bus Selector2 : BusSelector  OutputSignals=psi_rate_cmd
  Bus Selector3 : BusSelector  OutputSignals=phi,theta
  Demux : Demux  Outputs=3
  Euler To Angle Rate : FMT_Model_Lib/Math/Euler To Angle Rate
      settings: SourceProductName=FMT Toolbox
  Mux : Mux  Inputs=3
  Mux1 : Mux  Inputs=2
  Mux2 : Mux  Inputs=2
  Saturation : Saturate  UpperLimit=CONTROL_PARAM.MC_R_CMD_LIM  LowerLimit=-CONTROL_PARAM.MC_R_CMD_LIM
  Saturation1 : Saturate  UpperLimit=CONTROL_PARAM.MC_P_Q_CMD_LIM  LowerLimit=-CONTROL_PARAM.MC_P_Q_CMD_LIM
  Saturation2 : Saturate  UpperLimit=CONTROL_PARAM.MC_P_Q_CMD_LIM  LowerLimit=-CONTROL_PARAM.MC_P_Q_CMD_LIM
  rate_cmd_radPs : Outport
  wires:
  Bus Selector3/1 -> Mux2/1  "<phi>"
  Mux2/1 -> Euler To Angle Rate/1
  Bus Selector3/2 -> Mux2/2  "<theta>"
  Bus Selector2/1 -> Mux1/2  "<psi_rate_cmd>"
  Mux1/1 -> Euler To Angle Rate/2  "euler_rate"
  FMS_Out/1 -> Bus Selector2/1
  INS_Out/1 -> Bus Selector3/1
  Euler To Angle Rate/1 -> Demux/1  "ang_rate"
  euler_rate_cmd/1 -> Mux1/1
  Demux/1 -> Saturation1/1
  Demux/2 -> Saturation2/1
  Demux/3 -> Saturation/1
  Saturation1/1 -> Mux/1
  Mux/1 -> rate_cmd_radPs/1
  Saturation2/1 -> Mux/2
  Saturation/1 -> Mux/3

== system Controller/Controller/MC_Controller/Horizontal_Control/Attitude_Controller/Inner_Loop/Signal_Select ==
  note: mode:
      | 0: Unknown
      | 1: Mission
      | 2: Stablize
      | 3: Altitude Hold
      | 4: Attitude Mode
      | 5: Acro Mode
  FMS_Out : Inport
  rate_cmd_radPs : Inport  Port=2
  Bus Selector : BusSelector  OutputSignals=ctrl_mode
  Bus Selector1 : BusSelector  OutputSignals=p_cmd,q_cmd,r_cmd
  Compare To Constant : simulink/Logic and Bit Operations/Compare To Constant  relop===  const=uint8(ControlMode.Acro)  OutDataTypeStr=boolean
  Compare To Constant1 : simulink/Logic and Bit Operations/Compare To Constant  relop===  const=uint8(ControlMode.Offboard)  OutDataTypeStr=boolean
  Mux : Mux  Inputs=3
  Offboard_Signal_Select : Subsystem
  Switch : Switch  Criteria=u2 > Threshold
  Switch1 : Switch  Criteria=u2 > Threshold
  out : Outport
  wires:
  FMS_Out/1 -> Bus Selector/1, Offboard_Signal_Select/1(FMS_Out), Bus Selector1/1
  Switch/1 -> out/1
  Bus Selector/1 -> Compare To Constant1/1, Compare To Constant/1  "<ctrl_mode>"
  Compare To Constant/1 -> Switch/2
  Bus Selector1/1 -> Mux/1  "<p_cmd>"
  Bus Selector1/2 -> Mux/2  "<q_cmd>"
  Bus Selector1/3 -> Mux/3  "<r_cmd>"
  Mux/1 -> Switch/1
  rate_cmd_radPs/1 -> Switch1/3, Offboard_Signal_Select/2(rate_cmd_in)
  Switch1/1 -> Switch/3
  Offboard_Signal_Select/1(rate_cmd_radPs) -> Switch1/1
  Compare To Constant1/1 -> Switch1/2

== system Controller/Controller/MC_Controller/Horizontal_Control/Attitude_Controller/Outter_Loop/Attitude_Controller ==
  att_cmd_rad : Inport
  INS_Out : Inport  Port=2
  Error : Subsystem
  Sqrt_Root_Controller : Subsystem
  euler_rate_cmd_radPs : Outport
  wires:
  INS_Out/1 -> Error/2(INS_Out)
  Sqrt_Root_Controller/1(euler_rate_cmd_radPs) -> euler_rate_cmd_radPs/1
  att_cmd_rad/1 -> Error/1(att_cmd)
  Error/1(euler_err_rad) -> Sqrt_Root_Controller/1(euler_err_rad)

== system Controller/Controller/MC_Controller/Horizontal_Control/Attitude_Controller/Outter_Loop/Signal_Select ==
  note: mode:
      | 0: Unknown
      | 1: Mission
      | 2: Position
      | 3: Altitude Hold
      | 4: Manual Mode
      | 5: Acro Mode
      | 6: Offboard
  att_cmd_rad : Inport
  FMS_Out : Inport  Port=2
  Bus Selector : BusSelector  OutputSignals=ctrl_mode
  Bus Selector1 : BusSelector  OutputSignals=phi_cmd,theta_cmd
  Compare To Constant : simulink/Logic and Bit Operations/Compare To Constant  relop===  const=uint8([ControlMode.Stabilize, ControlMode.ALTCTL])  OutDataTypeStr=boolean
  Compare To Constant1 : simulink/Logic and Bit Operations/Compare To Constant  relop===  const=uint8(ControlMode.Offboard)  OutDataTypeStr=boolean
  Logical Operator : Logic  Operator=OR  Inputs=1  AllPortsSameDT=off  OutDataTypeStr=boolean
  Mux : Mux  Inputs=2
  Offboard_Signal_Select : Subsystem
  Switch : Switch  Criteria=u2 > Threshold
  Switch1 : Switch  Criteria=u2 > Threshold
  out : Outport
  wires:
  Compare To Constant/1 -> Logical Operator/1
  Bus Selector1/2 -> Mux/2  "<theta_cmd>"
  Bus Selector1/1 -> Mux/1  "<phi_cmd>"
  Bus Selector/1 -> Compare To Constant1/1, Compare To Constant/1  "<ctrl_mode>"
  FMS_Out/1 -> Bus Selector/1, Bus Selector1/1, Offboard_Signal_Select/1(FMS_Out)
  Mux/1 -> Switch/1
  Switch/1 -> out/1
  Logical Operator/1 -> Switch/2
  Switch1/1 -> Switch/3
  Compare To Constant1/1 -> Switch1/2
  Offboard_Signal_Select/1(att_cmd_rad) -> Switch1/1
  att_cmd_rad/1 -> Offboard_Signal_Select/2(att_cmd_in), Switch1/3

== system Controller/Controller/MC_Controller/Horizontal_Control/Velocity_Controller/Error/Bus_Select ==
  INS_Out : Inport
  Bus Selector1 : BusSelector  OutputSignals=vn,ve
  Bus Selector2 : BusSelector  OutputSignals=psi
  Constant : Constant  Value=0  OutDataTypeStr=single
  Multiply : Product  Multiplication=Matrix(*)
  Mux2 : Mux  Inputs=3
  Psi To DCM : FMT_Model_Lib/Transformation/Psi To DCM
      settings: SourceProductName=FMT Toolbox
  Selector : Selector  InputPortWidth=3  IndexOptions=Index vector (dialog)  Indices=[1 2]  OutputSizes=1
  uv_est_C_mPs : Outport
  wires:
  Psi To DCM/1 -> Multiply/1
  Bus Selector2/1 -> Psi To DCM/1  "<psi>"
  Constant/1 -> Mux2/3  "<velD>"
  Mux2/1 -> Multiply/2
  Bus Selector1/2 -> Mux2/2  "<ve>"
  Bus Selector1/1 -> Mux2/1  "<vn>"
  INS_Out/1 -> Bus Selector2/1, Bus Selector1/1
  Multiply/1 -> Selector/1
  Selector/1 -> uv_est_C_mPs/1

== system Controller/Controller/MC_Controller/Horizontal_Control/Velocity_Controller/Error/TD ==
  v : Inport
  Integrator : DiscreteIntegrator  SampleTime=-1  ICPrevOutput=DiscIntNeverNeededParam  ICPrevScaledInput=DiscIntNeverNeededParam
  Integrator1 : DiscreteIntegrator  SampleTime=-1  ICPrevOutput=DiscIntNeverNeededParam  ICPrevScaledInput=DiscIntNeverNeededParam
  Subtract : Sum  Inputs=+-
  "fhan " : Subsystem  mask{r0=8*9.806, h0=0.1}
      mask DialogControl ParameterGroupVar Prompt: fhan(v1,v2,r0,h0)
  v1 : Outport
  wires:
  Integrator1/1 -> v1/1, Subtract/1
  v/1 -> Subtract/2
  Integrator/1 -> "fhan "/2(v2), Integrator1/1  "v2"
  Subtract/1 -> "fhan "/1(v1)
  "fhan "/1(fhan) -> Integrator/1

== system Controller/Controller/MC_Controller/Horizontal_Control/Velocity_Controller/PID_Controller/D_Control ==
  err : Inport
  reset : Inport  Port=2
  DT Filter : FMT_Model_Lib/Filter/DT Filter  fc=10
      settings: SourceProductName=FMT Toolbox
  Multiply : Product  OutDataTypeStr=Inherit: Same as first input
  Saturation : Saturate  UpperLimit=max_d  LowerLimit=min_d
  kd : Constant  Value=kd  OutDataTypeStr=single
  d_out : Outport
  wires:
  err/1 -> DT Filter/1
  kd/1 -> Multiply/1
  Multiply/1 -> Saturation/1
  Saturation/1 -> d_out/1
  reset/1 -> DT Filter/2
  DT Filter/1 -> Multiply/2

== system Controller/Controller/MC_Controller/Horizontal_Control/Velocity_Controller/PID_Controller/I_Control ==
  err : Inport
  reset : Inport  Port=2
  Constant : Constant  Value=0  OutDataTypeStr=single
  Discrete-Time Integrator : DiscreteIntegrator  ExternalReset=level  InitialConditionSource=external  SampleTime=-1  LimitOutput=on  UpperSaturationLimit=max_i  LowerSaturationLimit=min_i  ICPrevOutput=DiscIntNeverNeededParam  ICPrevScaledInput=DiscIntNeverNeededParam
  Multiply : Product  OutDataTypeStr=Inherit: Same as first input
  ki : Constant  Value=ki  OutDataTypeStr=single
  i_out : Outport
  wires:
  err/1 -> Multiply/2
  Multiply/1 -> Discrete-Time Integrator/1
  reset/1 -> Discrete-Time Integrator/2
  Constant/1 -> Discrete-Time Integrator/3
  Discrete-Time Integrator/1 -> i_out/1
  ki/1 -> Multiply/1

== system Controller/Controller/MC_Controller/Horizontal_Control/Velocity_Controller/PID_Controller/P_Control ==
  err : Inport
  Multiply : Product  OutDataTypeStr=Inherit: Same as first input
  kp : Constant  Value=kp  OutDataTypeStr=single
  p_out : Outport
  wires:
  err/1 -> Multiply/2
  kp/1 -> Multiply/1
  Multiply/1 -> p_out/1

== system Controller/Controller/MC_Controller/Horizontal_Control/Velocity_Controller/Signal_Select/Offboard_Signal_Select ==
  FMS_Out : Inport
  acc_cmd_in : Inport  Port=2
  Bus Selector1 : BusSelector  OutputSignals=cmd_mask
  Bus Selector2 : BusSelector  OutputSignals=ax_cmd,ay_cmd
  Compare To Zero : simulink/Logic and Bit Operations/Compare To Zero  relop=>  OutDataTypeStr=boolean
  Compare To Zero2 : simulink/Logic and Bit Operations/Compare To Zero  relop=>  OutDataTypeStr=boolean
  Multiply2 : Product
  Multiply3 : Product
  Mux : Mux  Inputs=2
  Mux1 : Mux  Inputs=2
  Mux2 : Mux  Inputs=2
  Sum1 : Sum  Inputs=|++
  cmd_ax valid : simulink/Logic and Bit Operations/Bitwise Operator  logicop=AND  UseBitMask=on  BitMask=bin2dec('1000000000')  BitMaskRealWorld=Stored Integer
  cmd_ay valid : simulink/Logic and Bit Operations/Bitwise Operator  logicop=AND  UseBitMask=on  BitMask=bin2dec('10000000000')  BitMaskRealWorld=Stored Integer
  cmd_u valid : simulink/Logic and Bit Operations/Bitwise Operator  logicop=AND  UseBitMask=on  BitMask=bin2dec('1000000')  BitMaskRealWorld=Stored Integer
  cmd_v valid : simulink/Logic and Bit Operations/Bitwise Operator  logicop=AND  UseBitMask=on  BitMask=bin2dec('10000000')  BitMaskRealWorld=Stored Integer
  acc_cmd : Outport
  wires:
  Multiply2/1 -> Sum1/2
  FMS_Out/1 -> Bus Selector2/1, Bus Selector1/1
  Bus Selector1/1 -> cmd_v valid/1, cmd_u valid/1, cmd_ay valid/1, cmd_ax valid/1  "<cmd_mask>"
  Multiply3/1 -> Sum1/1
  cmd_u valid/1 -> Mux1/1
  cmd_v valid/1 -> Mux1/2
  Mux1/1 -> Compare To Zero/1
  acc_cmd_in/1 -> Multiply2/2
  Compare To Zero/1 -> Multiply2/1
  Bus Selector2/1 -> Mux/1  "<ax_cmd>"
  cmd_ax valid/1 -> Mux2/1
  cmd_ay valid/1 -> Mux2/2
  Mux2/1 -> Compare To Zero2/1
  Compare To Zero2/1 -> Multiply3/2
  Bus Selector2/2 -> Mux/2  "<ay_cmd>"
  Mux/1 -> Multiply3/1
  Sum1/1 -> acc_cmd/1

== system Controller/Controller/MC_Controller/Vertical_Control/Veloxity_Z_Controller/Error/TD ==
  v : Inport
  Integrator : DiscreteIntegrator  SampleTime=-1  ICPrevOutput=DiscIntNeverNeededParam  ICPrevScaledInput=DiscIntNeverNeededParam
  Integrator1 : DiscreteIntegrator  SampleTime=-1  ICPrevOutput=DiscIntNeverNeededParam  ICPrevScaledInput=DiscIntNeverNeededParam
  Subtract : Sum  Inputs=+-
  "fhan " : Subsystem  mask{r0=8*9.806, h0=0.05}
      mask DialogControl ParameterGroupVar Prompt: fhan(v1,v2,r0,h0)
  v1 : Outport
  wires:
  Integrator1/1 -> v1/1, Subtract/1
  v/1 -> Subtract/2
  Integrator/1 -> "fhan "/2(v2), Integrator1/1  "v2"
  Subtract/1 -> "fhan "/1(v1)
  "fhan "/1(fhan) -> Integrator/1

== system Controller/Controller/MC_Controller/Vertical_Control/Veloxity_Z_Controller/PID_Controller/D_Control ==
  err : Inport
  reset : Inport  Port=2
  DT Filter : FMT_Model_Lib/Filter/DT Filter  fc=10
      settings: SourceProductName=FMT Toolbox
  Multiply : Product  OutDataTypeStr=Inherit: Same as first input
  Saturation : Saturate  UpperLimit=max_d  LowerLimit=min_d
  kd : Constant  Value=kd  OutDataTypeStr=single
  d_out : Outport
  wires:
  err/1 -> DT Filter/1
  kd/1 -> Multiply/1
  Multiply/1 -> Saturation/1
  Saturation/1 -> d_out/1
  reset/1 -> DT Filter/2
  DT Filter/1 -> Multiply/2

== system Controller/Controller/MC_Controller/Vertical_Control/Veloxity_Z_Controller/PID_Controller/I_Control ==
  err : Inport
  reset : Inport  Port=2
  Constant : Constant  Value=min_i  OutDataTypeStr=single
  Discrete-Time Integrator : DiscreteIntegrator  ExternalReset=level  InitialConditionSource=external  SampleTime=-1  LimitOutput=on  UpperSaturationLimit=max_i  LowerSaturationLimit=min_i  ICPrevOutput=DiscIntNeverNeededParam  ICPrevScaledInput=DiscIntNeverNeededParam
  Multiply : Product  OutDataTypeStr=Inherit: Same as first input
  ki : Constant  Value=ki  OutDataTypeStr=single
  i_out : Outport
  wires:
  err/1 -> Multiply/2
  Multiply/1 -> Discrete-Time Integrator/1
  reset/1 -> Discrete-Time Integrator/2
  Constant/1 -> Discrete-Time Integrator/3
  Discrete-Time Integrator/1 -> i_out/1
  ki/1 -> Multiply/1

== system Controller/Controller/MC_Controller/Vertical_Control/Veloxity_Z_Controller/PID_Controller/P_Control ==
  err : Inport
  Multiply : Product  OutDataTypeStr=Inherit: Same as first input
  kp : Constant  Value=kp  OutDataTypeStr=single
  p_out : Outport
  wires:
  err/1 -> Multiply/2
  kp/1 -> Multiply/1
  Multiply/1 -> p_out/1

== system Controller/Controller/VTOL_Control_Allocation/VTOL_Control_Allocation/VTOL1/FW_Control_Allocation/FW_Effective_Matrix ==
  Constant1 : Constant  Value=CONTROL_PARAM.FW_ROLL_EFFC*CONTROL_PARAM.FW_AILERON1_DIR  OutDataTypeStr=single
  Constant{3..6,8..11} (8 alike) : Constant  Value=0  OutDataTypeStr=single
  Constant12 : Constant  Value=CONTROL_PARAM.FW_YAW_EFFC*CONTROL_PARAM.FW_RUDDER_DIR  OutDataTypeStr=single
  Constant2 : Constant  Value=CONTROL_PARAM.FW_ROLL_EFFC*CONTROL_PARAM.FW_AILERON2_DIR  OutDataTypeStr=single
  Constant7 : Constant  Value=CONTROL_PARAM.FW_PITCH_EFFC*CONTROL_PARAM.FW_ELEVATOR_DIR  OutDataTypeStr=single
  Matrix Concatenate : Concatenate  NumInputs=3  Mode=Multidimensional array  ConcatenateDimension=2
  Vector Concatenate : Concatenate  NumInputs=4
  Vector Concatenate1 : Concatenate  NumInputs=4
  Vector Concatenate2 : Concatenate  NumInputs=4
  EffecMat : Outport
  wires:
  Constant7/1 -> Vector Concatenate1/3
  Constant8/1 -> Vector Concatenate1/4
  Constant9/1 -> Vector Concatenate2/1
  Constant12/1 -> Vector Concatenate2/4
  Constant3/1 -> Vector Concatenate/3
  Vector Concatenate/1 -> Matrix Concatenate/1
  Matrix Concatenate/1 -> EffecMat/1
  Constant2/1 -> Vector Concatenate/2
  Constant11/1 -> Vector Concatenate2/3
  Constant10/1 -> Vector Concatenate2/2
  Constant1/1 -> Vector Concatenate/1
  Vector Concatenate2/1 -> Matrix Concatenate/3
  Constant4/1 -> Vector Concatenate/4
  Vector Concatenate1/1 -> Matrix Concatenate/2
  Constant5/1 -> Vector Concatenate1/1
  Constant6/1 -> Vector Concatenate1/2

== system Controller/Controller/VTOL_Control_Allocation/VTOL_Control_Allocation/VTOL1/FW_Control_Allocation/Signal_Select ==
  throttle_cmd_in : Inport
  FMS_Out : Inport  Port=2
  Bus Selector1 : BusSelector  OutputSignals=throttle_cmd,ctrl_mode
  Compare To Constant : simulink/Logic and Bit Operations/Compare To Constant  relop=<=  const=uint8(ControlMode.Stabilize)  OutDataTypeStr=boolean
  Switch : Switch  Criteria=u2 > Threshold
  throttle_cmd : Outport
  wires:
  Compare To Constant/1 -> Switch/2
  throttle_cmd_in/1 -> Switch/3  "ff6"
  Bus Selector1/2 -> Compare To Constant/1  "<ctrl_mode>"
  Bus Selector1/1 -> Switch/1  "<throttle_cmd>"
  FMS_Out/1 -> Bus Selector1/1
  Switch/1 -> throttle_cmd/1

== system Controller/Controller/VTOL_Control_Allocation/VTOL_Control_Allocation/VTOL1/FW_Control_Allocation/fw_throttle_mapping ==
  thrust_cmd : Inport
  Constant1 : Constant  Value=1000  OutDataTypeStr=uint32
  Data Type Conversion : DataTypeConversion  OutDataTypeStr=uint16
  Gain1 : Gain  Gain=1000  OutDataTypeStr=uint32
  Sum1 : Sum  Inputs=|++
  throttle_cmd : Outport
  wires:
  Sum1/1 -> Data Type Conversion/1
  thrust_cmd/1 -> Gain1/1
  Data Type Conversion/1 -> throttle_cmd/1
  Constant1/1 -> Sum1/2
  Gain1/1 -> Sum1/1
